simulink model "interpolation_nD_TestGen56"  (R2017b)
settings: Solver=FixedStepDiscrete  StartTime=0.0  StopTime=10.0  RelTol=1e-3
undefined symbols (not defined in the file): Block_TestLib, enable_trigger
settings Model: Creator=ktrinh  LastModifiedBy=ktrinh
settings DebuggingCC: ParameterOverflowMsg=none

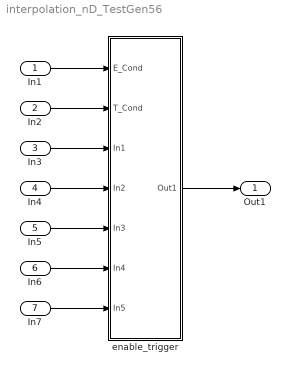
== system interpolation_nD_TestGen56 ==
  In1 : Inport
  In2 : Inport  Port=2
  In3 : Inport  Port=3  OutDataTypeStr=Bus: kfBus  BusOutputAsStruct=on
  In4 : Inport  Port=4  OutDataTypeStr=Bus: kfBus  BusOutputAsStruct=on
  In5 : Inport  Port=5  OutDataTypeStr=Bus: kfBus  BusOutputAsStruct=on
  In6 : Inport  Port=6
  In7 : Inport  Port=7
  enable_trigger : Subsystem  AncestorBlock=Block_TestLib/enable_trigger
  Out1 : Outport
  wires:
  In1/1 -> enable_trigger/1(E_Cond)
  In2/1 -> enable_trigger/2(T_Cond)
  In3/1 -> enable_trigger/3(In1)
  In4/1 -> enable_trigger/4(In2)
  In5/1 -> enable_trigger/5(In3)
  In6/1 -> enable_trigger/6(In4)
  In7/1 -> enable_trigger/7(In5)
  enable_trigger/1(Out1) -> Out1/1

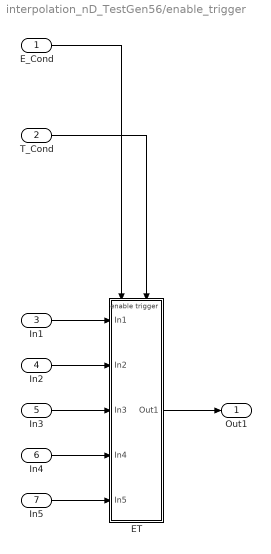
== system interpolation_nD_TestGen56/enable_trigger ==
  E_Cond : Inport  OutDataTypeStr=boolean
  T_Cond : Inport  Port=2  OutDataTypeStr=boolean
  In1 : Inport  Port=3  OutDataTypeStr=Bus: kfBus  BusOutputAsStruct=on
  In2 : Inport  Port=4  OutDataTypeStr=Bus: kfBus  BusOutputAsStruct=on
  In3 : Inport  Port=5  OutDataTypeStr=Bus: kfBus  BusOutputAsStruct=on
  In4 : Inport  Port=6
  In5 : Inport  Port=7
  ET : Subsystem  TreatAsAtomicUnit=on
  Out1 : Outport
  wires:
  T_Cond/1 -> ET/Trigger
  E_Cond/1 -> ET/Enable
  In1/1 -> ET/1(In1)
  In2/1 -> ET/2(In2)
  In3/1 -> ET/3(In3)
  In4/1 -> ET/4(In4)
  In5/1 -> ET/5(In5)
  ET/1(Out1) -> Out1/1

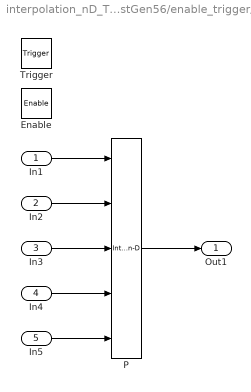
== system interpolation_nD_TestGen56/enable_trigger/ET ==
  In1 : Inport  OutMin=0  OutMax=2  OutDataTypeStr=Bus: kfBus  PortDimensions=1  BusOutputAsStruct=on
  In2 : Inport  Port=2  OutMin=0  OutMax=5  OutDataTypeStr=Bus: kfBus  BusOutputAsStruct=on
  In3 : Inport  Port=3  OutMin=0  OutMax=3  OutDataTypeStr=Bus: kfBus  BusOutputAsStruct=on
  In4 : Inport  Port=4  OutMin=0  OutMax=2
  In5 : Inport  Port=5  PortDimensions=[2 5 3 2]
  Enable : EnablePort
  Trigger : TriggerPort  VariantControl=Variant
  P : Interpolation_n-D  InitFcn=|  NumberOfTableDimensions=4  TableSource=Input port  InterpMethod=Flat  ExtrapMethod=Clip  RequireIndexFractionAsBus=on  NumSelectionDims=1  OutDataTypeStr=int16  InternalRulePriority=Speed  RndMeth=Ceiling  IntermediateResultsDataTypeStr=double
      | elems(1) = Simulink.BusElement;
      | elems(1).Name = 'Index';
      | elems(1).DataType = 'int8';
      | elems(2) = Simulink.BusElement;
      | elems(2).Name = 'Fraction';
      | elems(2).DataType = 'double';
      | kfBus = Simulink.Bus;
      | kfBus.Elements = elems;
      | clear elems;
      | assignin('base', 'kfBus', kfBus);
      settings: InputPortMap=u0,u1,u2,u3,p2
  Out1 : Outport
  wires:
  In1/1 -> P/1
  In2/1 -> P/2
  In3/1 -> P/3
  In4/1 -> P/4
  In5/1 -> P/5
  P/1 -> Out1/1
